simulink model "Position"  (R2016a)
settings: Solver=ode2  StartTime=0.0  StopTime=10.0  FixedStep=sample_time  RelTol=1e-3
InitFcn:
  | Parameters_quadrotor
  | Parameters_controllers
undefined symbols (not defined in the file): KB_X, KB_Y, KD_X, KD_Y, KI_X, KI_Y, KP_X, KP_Y, MAX_PITCH, MAX_ROLL, MIN_PITCH, MIN_ROLL, POS_N
libraries: simulink x2
settings Model: Creator=pela  LastModifiedBy=Mattia
settings DataIOCC: LimitDataPoints=on  SaveFormat=Array
settings HardwareCC: ProdBitPerPointer=32  ProdLargestAtomicInteger=Long  ProdLargestAtomicFloat=Double  ProdIntDivRoundTo=Undefined  ProdWordSize=32  ProdHWDeviceType=ARM Compatible->ARM Cortex
settings ModelReferenceCC: PropagateSignalLabelsOutOfModel=off
settings RTWCC: GenCodeOnly=on  GenerateReport=on  Toolchain=GNU gcc/g++ v4.4.x | gmake (64-bit Linux)  BuildConfiguration=Faster Runs  LaunchReport=on  TargetLang=C++
settings GRTTargetCC: MatFileLogging=off  MultiInstanceERTCode=on  CodeInterfacePackaging=C++ class  SupportNonFinite=off
settings ConfigComp: CovModelRefEnable=Off

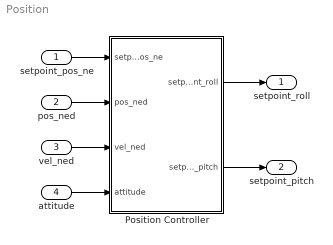
== system Position ==
  setpoint_pos_ne : Inport  PortDimensions=2
  pos_ned : Inport  Port=2  PortDimensions=2
  vel_ned : Inport  Port=3
  attitude : Inport  Port=4
  Position Controller : Subsystem
  setpoint_roll : Outport  PortDimensions=1
  setpoint_pitch : Outport  Port=2  PortDimensions=1
  wires:
  Position Controller/2(setpoint_pitch) -> setpoint_pitch/1
  setpoint_pos_ne/1 -> Position Controller/1(setpoint_pos_ne)
  Position Controller/1(setpoint_roll) -> setpoint_roll/1
  attitude/1 -> Position Controller/4(attitude)
  vel_ned/1 -> Position Controller/3(vel_ned)
  pos_ned/1 -> Position Controller/2(pos_ned)

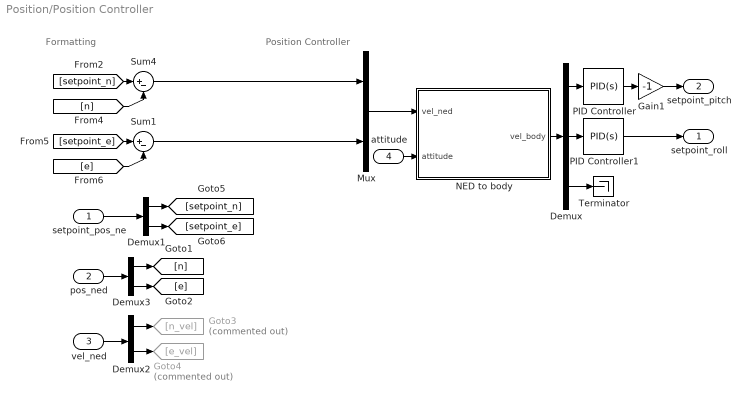
== system Position/Position Controller ==
  note: Formatting
  note: Position Controller
  setpoint_pos_ne : Inport  PortDimensions=2
  pos_ned : Inport  Port=2
  vel_ned : Inport  Port=3
  attitude : Inport  Port=4  PortDimensions=3
  Demux : Demux  Outputs=3
  Demux1 : Demux  Outputs=2
  Demux2 : Demux  Outputs=2
  Demux3 : Demux  Outputs=2
  Gain1 : Gain  Gain=-1
  Goto3 : Goto  Commented=on  GotoTag=n_vel
  Goto4 : Goto  Commented=on  GotoTag=e_vel
  Mux : Mux  Inputs=2
  NED to body : MATLAB Function  TreatAsAtomicUnit=on
  PID Controller : simulink/Continuous/PID Controller  Controller=PID  TimeDomain=Continuous-time  SampleTime=-1  IntegratorMethod=Forward Euler  FilterMethod=Trapezoidal  Form=Parallel  UseFilter=on  ControllerParametersSource=internal  P=KP_X  I=KI_X  D=KD_X  N=POS_N  InitialConditionSource=internal  InitialConditionForIntegrator=0  InitialConditionForFilter=0  ExternalReset=none  LimitOutput=on  UpperSaturationLimit=MAX_PITCH  LowerSaturationLimit=MIN_PITCH  LinearizeAsGain=on  AntiWindupMode=back-calculation  Kb=KB_X  TrackingMode=off  Kt=1  PParamMin=[]  PParamMax=[]  IParamMin=[]  IParamMax=[]  DParamMin=[]  DParamMax=[]  NParamMin=[]  NParamMax=[]  KbParamMin=[]  KbParamMax=[]  KtParamMin=[]  KtParamMax=[]  POutMin=[]  POutMax=[]  IOutMin=[]  IOutMax=[]  DOutMin=[]  DOutMax=[]  NOutMin=[]  NOutMax=[]  KbOutMin=[]  KbOutMax=[]  KtOutMin=[]  KtOutMax=[]  IntegratorOutMin=[]  IntegratorOutMax=[]  FilterOutMin=[]  FilterOutMax=[]  SumOutMin=[]  SumOutMax=[]  SumI1OutMin=[]  SumI1OutMax=[]  SumI2OutMin=[]  SumI2OutMax=[]  SumI3OutMin=[]  SumI3OutMax=[]  SumDOutMin=[]  SumDOutMax=[]  SaturationOutMin=[]  SaturationOutMax=[]  IntegratorContinuousStateAttributes=''  IntegratorStateMustResolveToSignalObject=off  IntegratorRTWStateStorageClass=Auto  FilterContinuousStateAttributes=''  FilterStateMustResolveToSignalObject=off  FilterRTWStateStorageClass=Auto  DifferentiatorICPrevScaledInput=0  DifferentiatorOutMin=[]  DifferentiatorOutMax=[]
  PID Controller1 : simulink/Continuous/PID Controller  Controller=PID  TimeDomain=Continuous-time  SampleTime=-1  IntegratorMethod=Forward Euler  FilterMethod=Trapezoidal  Form=Parallel  UseFilter=on  ControllerParametersSource=internal  P=KP_Y  I=KI_Y  D=KD_Y  N=POS_N  InitialConditionSource=internal  InitialConditionForIntegrator=0  InitialConditionForFilter=0  ExternalReset=none  LimitOutput=on  UpperSaturationLimit=MAX_ROLL  LowerSaturationLimit=MIN_ROLL  LinearizeAsGain=on  AntiWindupMode=back-calculation  Kb=KB_Y  TrackingMode=off  Kt=1  PParamMin=[]  PParamMax=[]  IParamMin=[]  IParamMax=[]  DParamMin=[]  DParamMax=[]  NParamMin=[]  NParamMax=[]  KbParamMin=[]  KbParamMax=[]  KtParamMin=[]  KtParamMax=[]  POutMin=[]  POutMax=[]  IOutMin=[]  IOutMax=[]  DOutMin=[]  DOutMax=[]  NOutMin=[]  NOutMax=[]  KbOutMin=[]  KbOutMax=[]  KtOutMin=[]  KtOutMax=[]  IntegratorOutMin=[]  IntegratorOutMax=[]  FilterOutMin=[]  FilterOutMax=[]  SumOutMin=[]  SumOutMax=[]  SumI1OutMin=[]  SumI1OutMax=[]  SumI2OutMin=[]  SumI2OutMax=[]  SumI3OutMin=[]  SumI3OutMax=[]  SumDOutMin=[]  SumDOutMax=[]  SaturationOutMin=[]  SaturationOutMax=[]  IntegratorContinuousStateAttributes=''  IntegratorStateMustResolveToSignalObject=off  IntegratorRTWStateStorageClass=Auto  FilterContinuousStateAttributes=''  FilterStateMustResolveToSignalObject=off  FilterRTWStateStorageClass=Auto  DifferentiatorICPrevScaledInput=0  DifferentiatorOutMin=[]  DifferentiatorOutMax=[]
  Sum1 : Sum  Inputs=|+-
  Sum4 : Sum  Inputs=|+-
  Terminator : Terminator
  setpoint_roll : Outport  PortDimensions=1
  setpoint_pitch : Outport  Port=2  PortDimensions=1
  wires:
  PID Controller1/1 -> setpoint_roll/1
  attitude/1 -> NED to body/2(attitude)
  pos_ned/1 -> Demux3/1
  Demux2/1 -> Goto3/1
  Demux2/2 -> Goto4/1
  vel_ned/1 -> Demux2/1
  PID Controller/1 -> Gain1/1
  Gain1/1 -> setpoint_pitch/1
  setpoint_pos_ne/1 -> Demux1/1
  Demux3/1 -> [n]
  Demux3/2 -> [e]
  Demux1/1 -> [setpoint_n]
  Demux1/2 -> [setpoint_e]
  [setpoint_n] -> Sum4/1
  [n] -> Sum4/2
  [setpoint_e] -> Sum1/1
  [e] -> Sum1/2
  Mux/1 -> NED to body/1(vel_ned)
  NED to body/1(vel_body) -> Demux/1
  Demux/1 -> PID Controller/1
  Demux/2 -> PID Controller1/1
  Sum4/1 -> Mux/1
  Sum1/1 -> Mux/2
  Demux/3 -> Terminator/1

== matlab function Position/Position Controller/NED to body ==
  data: vel_ned input; attitude input; vel_body output
function vel_body  = ned2body(vel_ned,attitude)

phi = 0;
theta = 0;
psi = attitude(3);

Vel_NED = [vel_ned(1) ;
    vel_ned(2) ;
    0];

Sphi = sin(phi);
Cphi = cos(phi);
Stheta = sin(theta);
Ctheta = cos(theta);
Spsi = sin(psi);
Cpsi = cos(psi);

ned2body = [        Ctheta*Cpsi               Ctheta*Spsi          -Stheta;
       Sphi*Stheta*Cpsi-Cphi*Spsi Sphi*Stheta*Spsi+Cphi*Cpsi Sphi*Ctheta ;
       Cphi*Stheta*Cpsi+Sphi*Spsi Cphi*Stheta*Spsi-Sphi*Cpsi Cphi*Ctheta];

vel_body = ned2body * Vel_NED;
